simulink library "alphaY_ul"  (R2020a)
settings: Solver=VariableStepAuto  StartTime=0.0  StopTime=10.0  RelTol=1e-3
settings Model: Creator=mcobb  LastModifiedBy=John Jr
settings DataIOCC: ReturnWorkspaceOutputs=off
settings DebuggingCC: ArithmeticOperatorsInVariantConditions=warning
settings SFSimCC: CustomCodeUndefinedFunction=UseInterfaceOnly

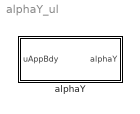
== system alphaY_ul ==
  alphaY : Subsystem  TreatAsAtomicUnit=on
      settings: MinAlgLoopOccurrences=on

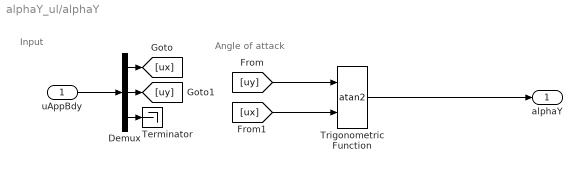
== system alphaY_ul/alphaY ==
  note: Angle of attack
  note: Input
  uAppBdy : Inport
  Demux : Demux  Outputs=3
  Terminator : Terminator
  Trigonometric Function : Trigonometry  Operator=atan2
  alphaY : Outport  VectorParamsAs1DForOutWhenUnconnected=off
  wires:
  uAppBdy/1 -> Demux/1
  Demux/1 -> [ux]
  Demux/2 -> [uy]
  Demux/3 -> Terminator/1
  Trigonometric Function/1 -> alphaY/1
  [uy] -> Trigonometric Function/1
  [ux] -> Trigonometric Function/2
